simulink model "ARAI_Academy"  (R2020a)
settings: Solver=FixedStepDiscrete  StartTime=0.0  StopTime=10.0  FixedStep=0.02  RelTol=1e-3
InitFcn:
  | mbd_s32k_consistency_checks(bdroot(gcs));
undefined symbols (not defined in the file): Cells_in_Series, LQFP, Temp_in_Series, ts
libraries: hdlsllib x280, mbd_s32k1xx_ec_toolbox x39, simulink x3
(part 2 of 3)

== system ARAI_Academy/Subsystem16/Subsystem12 ==
  In1 : Inport
  Data Type Conversion : DataTypeConversion  OutDataTypeStr=int16
  Demux : Demux  Outputs=8
  Mux : Mux  Inputs=8
  Subsystem : Subsystem
  Subsystem1 : Subsystem
  Subsystem2 : Subsystem
  Subsystem3 : Subsystem
  Subsystem4 : Subsystem
  Subsystem5 : Subsystem
  Subsystem7 : Subsystem
  Subsystem8 : Subsystem
  MO_CT_FLT : Outport
  wires:
  In1/1 -> Data Type Conversion/1
  Demux/1 -> Subsystem/1(u)
  Demux/2 -> Subsystem1/1(u)
  Demux/3 -> Subsystem2/1(u)
  Demux/4 -> Subsystem3/1(u)
  Demux/5 -> Subsystem4/1(u)
  Demux/6 -> Subsystem5/1(u)
  Demux/7 -> Subsystem7/1(u)
  Demux/8 -> Subsystem8/1(u)
  Subsystem/1(Out1) -> Mux/1
  Subsystem1/1(Out1) -> Mux/2
  Subsystem2/1(Out1) -> Mux/3
  Subsystem3/1(Out1) -> Mux/4
  Subsystem4/1(Out1) -> Mux/5
  Subsystem5/1(Out1) -> Mux/6
  Subsystem7/1(Out1) -> Mux/7
  Subsystem8/1(Out1) -> Mux/8
  Mux/1 -> MO_CT_FLT/1
  Data Type Conversion/1 -> Demux/1

== system ARAI_Academy/Subsystem17/Subsystem1 ==
  In1 : Inport
  Bit Slice : hdlsllib/Logic and Bit Operations/Bit Slice  lidx=15  ridx=8
      settings: SourceProductBaseCode=SL
  Bit Slice1 : hdlsllib/Logic and Bit Operations/Bit Slice  lidx=7  ridx=0
      settings: SourceProductBaseCode=SL
  Data Type Conversion : DataTypeConversion  OutDataTypeStr=uint16
  Mux : Mux  Inputs=2
  MO_MaxCellV : Outport
  wires:
  Data Type Conversion/1 -> Bit Slice/1, Bit Slice1/1
  Bit Slice/1 -> Mux/1
  Bit Slice1/1 -> Mux/2
  Mux/1 -> MO_MaxCellV/1  "MaxCellV"
  In1/1 -> Data Type Conversion/1

== system ARAI_Academy/Subsystem17/Subsystem9 ==
  HI_ICT_Raw : Inport
  Bit Slice : hdlsllib/Logic and Bit Operations/Bit Slice  lidx=15  ridx=8
      settings: SourceProductBaseCode=SL
  Bit Slice1 : hdlsllib/Logic and Bit Operations/Bit Slice  lidx=7  ridx=0
      settings: SourceProductBaseCode=SL
  Mux : Mux  Inputs=2
  MO_ICT : Outport
  wires:
  Mux/1 -> MO_ICT/1
  Bit Slice1/1 -> Mux/2
  HI_ICT_Raw/1 -> Bit Slice/1, Bit Slice1/1
  Bit Slice/1 -> Mux/1

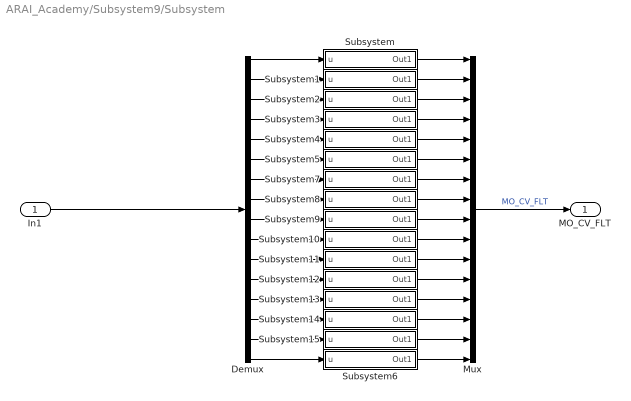
== system ARAI_Academy/Subsystem9/Subsystem ==
  In1 : Inport
  Demux : Demux  Outputs=16
  Mux : Mux  Inputs=16
  Subsystem : Subsystem
  Subsystem1 : Subsystem
  Subsystem10 : Subsystem
  Subsystem11 : Subsystem
  Subsystem12 : Subsystem
  Subsystem13 : Subsystem
  Subsystem14 : Subsystem
  Subsystem15 : Subsystem
  Subsystem2 : Subsystem
  Subsystem3 : Subsystem
  Subsystem4 : Subsystem
  Subsystem5 : Subsystem
  Subsystem6 : Subsystem
  Subsystem7 : Subsystem
  Subsystem8 : Subsystem
  Subsystem9 : Subsystem
  MO_CV_FLT : Outport
  wires:
  In1/1 -> Demux/1
  Demux/1 -> Subsystem/1(u)
  Demux/16 -> Subsystem6/1(u)
  Demux/2 -> Subsystem1/1(u)
  Demux/3 -> Subsystem2/1(u)
  Demux/4 -> Subsystem3/1(u)
  Demux/5 -> Subsystem4/1(u)
  Demux/6 -> Subsystem5/1(u)
  Demux/7 -> Subsystem7/1(u)
  Demux/8 -> Subsystem8/1(u)
  Demux/9 -> Subsystem9/1(u)
  Demux/10 -> Subsystem10/1(u)
  Demux/11 -> Subsystem11/1(u)
  Demux/12 -> Subsystem12/1(u)
  Demux/13 -> Subsystem13/1(u)
  Demux/14 -> Subsystem14/1(u)
  Demux/15 -> Subsystem15/1(u)
  Subsystem/1(Out1) -> Mux/1
  Subsystem1/1(Out1) -> Mux/2
  Subsystem2/1(Out1) -> Mux/3
  Subsystem3/1(Out1) -> Mux/4
  Subsystem4/1(Out1) -> Mux/5
  Subsystem5/1(Out1) -> Mux/6
  Subsystem7/1(Out1) -> Mux/7
  Subsystem8/1(Out1) -> Mux/8
  Subsystem9/1(Out1) -> Mux/9
  Subsystem10/1(Out1) -> Mux/10
  Subsystem11/1(Out1) -> Mux/11
  Subsystem12/1(Out1) -> Mux/12
  Subsystem13/1(Out1) -> Mux/13
  Subsystem14/1(Out1) -> Mux/14
  Subsystem15/1(Out1) -> Mux/15
  Subsystem6/1(Out1) -> Mux/16
  Mux/1 -> MO_CV_FLT/1  "MO_CV_FLT"

== system ARAI_Academy/TNS/ADC ==
  ADC_01 : Subsystem
  ADC_02 : Subsystem

== system ARAI_Academy/TNS/CAN ==
  CAN_01 : Subsystem

== system ARAI_Academy/TNS/I2C ==
  RTC/EEPROM : Subsystem

== system ARAI_Academy/TNS/System Outputs ==

== system ARAI_Academy/AFE_IN_SYS/If Action Subsystem/Subsystem ==
  Constant10 : Constant  Value=8  OutDataTypeStr=uint16  SampleTime=-1
  Constant11 : Constant  Value=32  OutDataTypeStr=uint32  SampleTime=-1
  Constant3 : Constant  Value=0x14  OutDataTypeStr=uint8  SampleTime=-1
  Constant8 : Constant  Value=true  OutDataTypeStr=Inherit: Inherit via back propagation  SampleTime=-1
  LPI2C_Master_Multi_Transfer : mbd_s32k1xx_ec_toolbox/Communication Blocks/I2C Blocks/LPI2C_Master_Multi_Transfer  instance=0  xfermode=Blocking  Timeout=3  delay_between_transfers=0  is10bit=off
  Out1 : Outport  PortDimensions=32
  wires:
  Constant10/1 -> LPI2C_Master_Multi_Transfer/3
  Constant3/1 -> LPI2C_Master_Multi_Transfer/1
  Constant8/1 -> LPI2C_Master_Multi_Transfer/2
  Constant11/1 -> LPI2C_Master_Multi_Transfer/4
  LPI2C_Master_Multi_Transfer/1 -> Out1/1

== system ARAI_Academy/AFE_IN_SYS/If Action Subsystem1/Subsystem ==
  Constant12 : Constant  Value=0x6A  OutDataTypeStr=uint8
  Constant13 : Constant  Value=true  OutDataTypeStr=Inherit: Inherit via back propagation
  Constant14 : Constant  Value=8  OutDataTypeStr=uint16
  Constant18 : Constant  Value=18  OutDataTypeStr=uint32
  LPI2C_Master_Multi_Transfer1 : mbd_s32k1xx_ec_toolbox/Communication Blocks/I2C Blocks/LPI2C_Master_Multi_Transfer  instance=0  xfermode=Blocking  Timeout=3  delay_between_transfers=0  is10bit=off
  Out1 : Outport  OutDataTypeStr=uint8  PortDimensions=18
  wires:
  Constant13/1 -> LPI2C_Master_Multi_Transfer1/2
  Constant18/1 -> LPI2C_Master_Multi_Transfer1/4
  LPI2C_Master_Multi_Transfer1/1 -> Out1/1
  Constant14/1 -> LPI2C_Master_Multi_Transfer1/3
  Constant12/1 -> LPI2C_Master_Multi_Transfer1/1

== system ARAI_Academy/AFE_IN_SYS/Subsystem1/Subsystem ==
  In1 : Inport  PortDimensions=2
  Bit Concat : hdlsllib/Logic and Bit Operations/Bit Concat  numInputs=2
  Demux : Demux  Outputs=2
  y : Outport
  wires:
  Demux/2 -> Bit Concat/2
  Demux/1 -> Bit Concat/1
  Bit Concat/1 -> y/1
  In1/1 -> Demux/1

== system ARAI_Academy/AFE_IN_SYS/Subsystem2/Subsystem ==
  In1 : Inport  PortDimensions=2
  Bit Concat : hdlsllib/Logic and Bit Operations/Bit Concat  numInputs=2
  Demux : Demux  Outputs=2
  y : Outport
  wires:
  Demux/2 -> Bit Concat/1
  Demux/1 -> Bit Concat/2
  Bit Concat/1 -> y/1
  In1/1 -> Demux/1

== system ARAI_Academy/AFE_IN_SYS/Subsystem3/Subsystem ==
  In1 : Inport  PortDimensions=2
  Bit Concat : hdlsllib/Logic and Bit Operations/Bit Concat  numInputs=2
  Demux : Demux  Outputs=2
  y : Outport
  wires:
  Demux/2 -> Bit Concat/1
  Demux/1 -> Bit Concat/2
  Bit Concat/1 -> y/1
  In1/1 -> Demux/1

== system ARAI_Academy/Subsystem10/Subsystem/Subsystem ==
  u : Inport
  Bit Slice : hdlsllib/Logic and Bit Operations/Bit Slice  lidx=15  ridx=8
      settings: SourceProductBaseCode=SL
  Bit Slice1 : hdlsllib/Logic and Bit Operations/Bit Slice  lidx=7  ridx=0
      settings: SourceProductBaseCode=SL
  Mux : Mux  Inputs=2
  Out1 : Outport
  wires:
  Bit Slice/1 -> Mux/1
  u/1 -> Bit Slice/1, Bit Slice1/1
  Bit Slice1/1 -> Mux/2
  Mux/1 -> Out1/1

== system ARAI_Academy/Subsystem10/Subsystem/Subsystem1 ==
  u : Inport
  Bit Slice : hdlsllib/Logic and Bit Operations/Bit Slice  lidx=15  ridx=8
      settings: SourceProductBaseCode=SL
  Bit Slice1 : hdlsllib/Logic and Bit Operations/Bit Slice  lidx=7  ridx=0
      settings: SourceProductBaseCode=SL
  Mux : Mux  Inputs=2
  Out1 : Outport
  wires:
  Bit Slice/1 -> Mux/1
  u/1 -> Bit Slice/1, Bit Slice1/1
  Bit Slice1/1 -> Mux/2
  Mux/1 -> Out1/1

== system ARAI_Academy/Subsystem10/Subsystem/Subsystem10 ==
  u : Inport
  Bit Slice : hdlsllib/Logic and Bit Operations/Bit Slice  lidx=15  ridx=8
      settings: SourceProductBaseCode=SL
  Bit Slice1 : hdlsllib/Logic and Bit Operations/Bit Slice  lidx=7  ridx=0
      settings: SourceProductBaseCode=SL
  Mux : Mux  Inputs=2
  Out1 : Outport
  wires:
  Bit Slice/1 -> Mux/1
  u/1 -> Bit Slice/1, Bit Slice1/1
  Bit Slice1/1 -> Mux/2
  Mux/1 -> Out1/1

== system ARAI_Academy/Subsystem10/Subsystem/Subsystem11 ==
  u : Inport
  Bit Slice : hdlsllib/Logic and Bit Operations/Bit Slice  lidx=15  ridx=8
      settings: SourceProductBaseCode=SL
  Bit Slice1 : hdlsllib/Logic and Bit Operations/Bit Slice  lidx=7  ridx=0
      settings: SourceProductBaseCode=SL
  Mux : Mux  Inputs=2
  Out1 : Outport
  wires:
  Mux/1 -> Out1/1
  Bit Slice1/1 -> Mux/2
  u/1 -> Bit Slice1/1, Bit Slice/1
  Bit Slice/1 -> Mux/1

== system ARAI_Academy/Subsystem10/Subsystem/Subsystem12 ==
  u : Inport
  Bit Slice : hdlsllib/Logic and Bit Operations/Bit Slice  lidx=15  ridx=8
      settings: SourceProductBaseCode=SL
  Bit Slice1 : hdlsllib/Logic and Bit Operations/Bit Slice  lidx=7  ridx=0
      settings: SourceProductBaseCode=SL
  Mux : Mux  Inputs=2
  Out1 : Outport
  wires:
  Bit Slice/1 -> Mux/1
  u/1 -> Bit Slice/1, Bit Slice1/1
  Bit Slice1/1 -> Mux/2
  Mux/1 -> Out1/1

== system ARAI_Academy/Subsystem10/Subsystem/Subsystem13 ==
  u : Inport
  Bit Slice : hdlsllib/Logic and Bit Operations/Bit Slice  lidx=15  ridx=8
      settings: SourceProductBaseCode=SL
  Bit Slice1 : hdlsllib/Logic and Bit Operations/Bit Slice  lidx=7  ridx=0
      settings: SourceProductBaseCode=SL
  Mux : Mux  Inputs=2
  Out1 : Outport
  wires:
  Mux/1 -> Out1/1
  Bit Slice1/1 -> Mux/2
  u/1 -> Bit Slice1/1, Bit Slice/1
  Bit Slice/1 -> Mux/1

== system ARAI_Academy/Subsystem10/Subsystem/Subsystem14 ==
  u : Inport
  Bit Slice : hdlsllib/Logic and Bit Operations/Bit Slice  lidx=15  ridx=8
      settings: SourceProductBaseCode=SL
  Bit Slice1 : hdlsllib/Logic and Bit Operations/Bit Slice  lidx=7  ridx=0
      settings: SourceProductBaseCode=SL
  Mux : Mux  Inputs=2
  Out1 : Outport
  wires:
  Bit Slice/1 -> Mux/1
  u/1 -> Bit Slice/1, Bit Slice1/1
  Bit Slice1/1 -> Mux/2
  Mux/1 -> Out1/1

== system ARAI_Academy/Subsystem10/Subsystem/Subsystem15 ==
  u : Inport
  Bit Slice : hdlsllib/Logic and Bit Operations/Bit Slice  lidx=15  ridx=8
      settings: SourceProductBaseCode=SL
  Bit Slice1 : hdlsllib/Logic and Bit Operations/Bit Slice  lidx=7  ridx=0
      settings: SourceProductBaseCode=SL
  Mux : Mux  Inputs=2
  Out1 : Outport
  wires:
  Mux/1 -> Out1/1
  Bit Slice1/1 -> Mux/2
  u/1 -> Bit Slice1/1, Bit Slice/1
  Bit Slice/1 -> Mux/1

== system ARAI_Academy/Subsystem10/Subsystem/Subsystem2 ==
  u : Inport
  Bit Slice : hdlsllib/Logic and Bit Operations/Bit Slice  lidx=15  ridx=8
      settings: SourceProductBaseCode=SL
  Bit Slice1 : hdlsllib/Logic and Bit Operations/Bit Slice  lidx=7  ridx=0
      settings: SourceProductBaseCode=SL
  Mux : Mux  Inputs=2
  Out1 : Outport
  wires:
  Bit Slice/1 -> Mux/1
  u/1 -> Bit Slice/1, Bit Slice1/1
  Bit Slice1/1 -> Mux/2
  Mux/1 -> Out1/1

== system ARAI_Academy/Subsystem10/Subsystem/Subsystem3 ==
  u : Inport
  Bit Slice : hdlsllib/Logic and Bit Operations/Bit Slice  lidx=15  ridx=8
      settings: SourceProductBaseCode=SL
  Bit Slice1 : hdlsllib/Logic and Bit Operations/Bit Slice  lidx=7  ridx=0
      settings: SourceProductBaseCode=SL
  Mux : Mux  Inputs=2
  Out1 : Outport
  wires:
  Bit Slice/1 -> Mux/1
  u/1 -> Bit Slice/1, Bit Slice1/1
  Bit Slice1/1 -> Mux/2
  Mux/1 -> Out1/1

== system ARAI_Academy/Subsystem10/Subsystem/Subsystem4 ==
  u : Inport
  Bit Slice : hdlsllib/Logic and Bit Operations/Bit Slice  lidx=15  ridx=8
      settings: SourceProductBaseCode=SL
  Bit Slice1 : hdlsllib/Logic and Bit Operations/Bit Slice  lidx=7  ridx=0
      settings: SourceProductBaseCode=SL
  Mux : Mux  Inputs=2
  Out1 : Outport
  wires:
  Bit Slice/1 -> Mux/1
  u/1 -> Bit Slice/1, Bit Slice1/1
  Bit Slice1/1 -> Mux/2
  Mux/1 -> Out1/1

== system ARAI_Academy/Subsystem10/Subsystem/Subsystem5 ==
  u : Inport
  Bit Slice : hdlsllib/Logic and Bit Operations/Bit Slice  lidx=15  ridx=8
      settings: SourceProductBaseCode=SL
  Bit Slice1 : hdlsllib/Logic and Bit Operations/Bit Slice  lidx=7  ridx=0
      settings: SourceProductBaseCode=SL
  Mux : Mux  Inputs=2
  Out1 : Outport
  wires:
  Bit Slice/1 -> Mux/1
  u/1 -> Bit Slice/1, Bit Slice1/1
  Bit Slice1/1 -> Mux/2
  Mux/1 -> Out1/1

== system ARAI_Academy/Subsystem10/Subsystem/Subsystem6 ==
  u : Inport
  Bit Slice : hdlsllib/Logic and Bit Operations/Bit Slice  lidx=15  ridx=8
      settings: SourceProductBaseCode=SL
  Bit Slice1 : hdlsllib/Logic and Bit Operations/Bit Slice  lidx=7  ridx=0
      settings: SourceProductBaseCode=SL
  Mux : Mux  Inputs=2
  Out1 : Outport
  wires:
  Bit Slice/1 -> Mux/1
  u/1 -> Bit Slice/1, Bit Slice1/1
  Bit Slice1/1 -> Mux/2
  Mux/1 -> Out1/1

== system ARAI_Academy/Subsystem10/Subsystem/Subsystem7 ==
  u : Inport
  Bit Slice : hdlsllib/Logic and Bit Operations/Bit Slice  lidx=15  ridx=8
      settings: SourceProductBaseCode=SL
  Bit Slice1 : hdlsllib/Logic and Bit Operations/Bit Slice  lidx=7  ridx=0
      settings: SourceProductBaseCode=SL
  Mux : Mux  Inputs=2
  Out1 : Outport
  wires:
  Mux/1 -> Out1/1
  Bit Slice1/1 -> Mux/2
  u/1 -> Bit Slice1/1, Bit Slice/1
  Bit Slice/1 -> Mux/1

== system ARAI_Academy/Subsystem10/Subsystem/Subsystem8 ==
  u : Inport
  Bit Slice : hdlsllib/Logic and Bit Operations/Bit Slice  lidx=15  ridx=8
      settings: SourceProductBaseCode=SL
  Bit Slice1 : hdlsllib/Logic and Bit Operations/Bit Slice  lidx=7  ridx=0
      settings: SourceProductBaseCode=SL
  Mux : Mux  Inputs=2
  Out1 : Outport
  wires:
  Bit Slice/1 -> Mux/1
  u/1 -> Bit Slice/1, Bit Slice1/1
  Bit Slice1/1 -> Mux/2
  Mux/1 -> Out1/1

== system ARAI_Academy/Subsystem10/Subsystem/Subsystem9 ==
  u : Inport
  Bit Slice : hdlsllib/Logic and Bit Operations/Bit Slice  lidx=15  ridx=8
      settings: SourceProductBaseCode=SL
  Bit Slice1 : hdlsllib/Logic and Bit Operations/Bit Slice  lidx=7  ridx=0
      settings: SourceProductBaseCode=SL
  Mux : Mux  Inputs=2
  Out1 : Outport
  wires:
  Mux/1 -> Out1/1
  Bit Slice1/1 -> Mux/2
  u/1 -> Bit Slice1/1, Bit Slice/1
  Bit Slice/1 -> Mux/1

== system ARAI_Academy/Subsystem11/Subsystem/Subsystem ==
  u : Inport
  Bit Slice : hdlsllib/Logic and Bit Operations/Bit Slice  lidx=15  ridx=8
      settings: SourceProductBaseCode=SL
  Bit Slice1 : hdlsllib/Logic and Bit Operations/Bit Slice  lidx=7  ridx=0
      settings: SourceProductBaseCode=SL
  Mux : Mux  Inputs=2
  Out1 : Outport
  wires:
  Bit Slice/1 -> Mux/1
  u/1 -> Bit Slice/1, Bit Slice1/1
  Bit Slice1/1 -> Mux/2
  Mux/1 -> Out1/1

== system ARAI_Academy/Subsystem11/Subsystem/Subsystem1 ==
  u : Inport
  Bit Slice : hdlsllib/Logic and Bit Operations/Bit Slice  lidx=15  ridx=8
      settings: SourceProductBaseCode=SL
  Bit Slice1 : hdlsllib/Logic and Bit Operations/Bit Slice  lidx=7  ridx=0
      settings: SourceProductBaseCode=SL
  Mux : Mux  Inputs=2
  Out1 : Outport
  wires:
  Bit Slice/1 -> Mux/1
  u/1 -> Bit Slice/1, Bit Slice1/1
  Bit Slice1/1 -> Mux/2
  Mux/1 -> Out1/1

== system ARAI_Academy/Subsystem11/Subsystem/Subsystem10 ==
  u : Inport
  Bit Slice : hdlsllib/Logic and Bit Operations/Bit Slice  lidx=15  ridx=8
      settings: SourceProductBaseCode=SL
  Bit Slice1 : hdlsllib/Logic and Bit Operations/Bit Slice  lidx=7  ridx=0
      settings: SourceProductBaseCode=SL
  Mux : Mux  Inputs=2
  Out1 : Outport
  wires:
  Bit Slice/1 -> Mux/1
  u/1 -> Bit Slice/1, Bit Slice1/1
  Bit Slice1/1 -> Mux/2
  Mux/1 -> Out1/1

== system ARAI_Academy/Subsystem11/Subsystem/Subsystem11 ==
  u : Inport
  Bit Slice : hdlsllib/Logic and Bit Operations/Bit Slice  lidx=15  ridx=8
      settings: SourceProductBaseCode=SL
  Bit Slice1 : hdlsllib/Logic and Bit Operations/Bit Slice  lidx=7  ridx=0
      settings: SourceProductBaseCode=SL
  Mux : Mux  Inputs=2
  Out1 : Outport
  wires:
  Mux/1 -> Out1/1
  Bit Slice1/1 -> Mux/2
  u/1 -> Bit Slice1/1, Bit Slice/1
  Bit Slice/1 -> Mux/1

== system ARAI_Academy/Subsystem11/Subsystem/Subsystem12 ==
  u : Inport
  Bit Slice : hdlsllib/Logic and Bit Operations/Bit Slice  lidx=15  ridx=8
      settings: SourceProductBaseCode=SL
  Bit Slice1 : hdlsllib/Logic and Bit Operations/Bit Slice  lidx=7  ridx=0
      settings: SourceProductBaseCode=SL
  Mux : Mux  Inputs=2
  Out1 : Outport
  wires:
  Bit Slice/1 -> Mux/1
  u/1 -> Bit Slice/1, Bit Slice1/1
  Bit Slice1/1 -> Mux/2
  Mux/1 -> Out1/1

== system ARAI_Academy/Subsystem11/Subsystem/Subsystem13 ==
  u : Inport
  Bit Slice : hdlsllib/Logic and Bit Operations/Bit Slice  lidx=15  ridx=8
      settings: SourceProductBaseCode=SL
  Bit Slice1 : hdlsllib/Logic and Bit Operations/Bit Slice  lidx=7  ridx=0
      settings: SourceProductBaseCode=SL
  Mux : Mux  Inputs=2
  Out1 : Outport
  wires:
  Mux/1 -> Out1/1
  Bit Slice1/1 -> Mux/2
  u/1 -> Bit Slice1/1, Bit Slice/1
  Bit Slice/1 -> Mux/1

== system ARAI_Academy/Subsystem11/Subsystem/Subsystem14 ==
  u : Inport
  Bit Slice : hdlsllib/Logic and Bit Operations/Bit Slice  lidx=15  ridx=8
      settings: SourceProductBaseCode=SL
  Bit Slice1 : hdlsllib/Logic and Bit Operations/Bit Slice  lidx=7  ridx=0
      settings: SourceProductBaseCode=SL
  Mux : Mux  Inputs=2
  Out1 : Outport
  wires:
  Bit Slice/1 -> Mux/1
  u/1 -> Bit Slice/1, Bit Slice1/1
  Bit Slice1/1 -> Mux/2
  Mux/1 -> Out1/1

== system ARAI_Academy/Subsystem11/Subsystem/Subsystem15 ==
  u : Inport
  Bit Slice : hdlsllib/Logic and Bit Operations/Bit Slice  lidx=15  ridx=8
      settings: SourceProductBaseCode=SL
  Bit Slice1 : hdlsllib/Logic and Bit Operations/Bit Slice  lidx=7  ridx=0
      settings: SourceProductBaseCode=SL
  Mux : Mux  Inputs=2
  Out1 : Outport
  wires:
  Mux/1 -> Out1/1
  Bit Slice1/1 -> Mux/2
  u/1 -> Bit Slice1/1, Bit Slice/1
  Bit Slice/1 -> Mux/1

== system ARAI_Academy/Subsystem11/Subsystem/Subsystem2 ==
  u : Inport
  Bit Slice : hdlsllib/Logic and Bit Operations/Bit Slice  lidx=15  ridx=8
      settings: SourceProductBaseCode=SL
  Bit Slice1 : hdlsllib/Logic and Bit Operations/Bit Slice  lidx=7  ridx=0
      settings: SourceProductBaseCode=SL
  Mux : Mux  Inputs=2
  Out1 : Outport
  wires:
  Bit Slice/1 -> Mux/1
  u/1 -> Bit Slice/1, Bit Slice1/1
  Bit Slice1/1 -> Mux/2
  Mux/1 -> Out1/1

== system ARAI_Academy/Subsystem11/Subsystem/Subsystem3 ==
  u : Inport
  Bit Slice : hdlsllib/Logic and Bit Operations/Bit Slice  lidx=15  ridx=8
      settings: SourceProductBaseCode=SL
  Bit Slice1 : hdlsllib/Logic and Bit Operations/Bit Slice  lidx=7  ridx=0
      settings: SourceProductBaseCode=SL
  Mux : Mux  Inputs=2
  Out1 : Outport
  wires:
  Bit Slice/1 -> Mux/1
  u/1 -> Bit Slice/1, Bit Slice1/1
  Bit Slice1/1 -> Mux/2
  Mux/1 -> Out1/1

== system ARAI_Academy/Subsystem11/Subsystem/Subsystem4 ==
  u : Inport
  Bit Slice : hdlsllib/Logic and Bit Operations/Bit Slice  lidx=15  ridx=8
      settings: SourceProductBaseCode=SL
  Bit Slice1 : hdlsllib/Logic and Bit Operations/Bit Slice  lidx=7  ridx=0
      settings: SourceProductBaseCode=SL
  Mux : Mux  Inputs=2
  Out1 : Outport
  wires:
  Bit Slice/1 -> Mux/1
  u/1 -> Bit Slice/1, Bit Slice1/1
  Bit Slice1/1 -> Mux/2
  Mux/1 -> Out1/1

== system ARAI_Academy/Subsystem11/Subsystem/Subsystem5 ==
  u : Inport
  Bit Slice : hdlsllib/Logic and Bit Operations/Bit Slice  lidx=15  ridx=8
      settings: SourceProductBaseCode=SL
  Bit Slice1 : hdlsllib/Logic and Bit Operations/Bit Slice  lidx=7  ridx=0
      settings: SourceProductBaseCode=SL
  Mux : Mux  Inputs=2
  Out1 : Outport
  wires:
  Bit Slice/1 -> Mux/1
  u/1 -> Bit Slice/1, Bit Slice1/1
  Bit Slice1/1 -> Mux/2
  Mux/1 -> Out1/1

== system ARAI_Academy/Subsystem11/Subsystem/Subsystem6 ==
  u : Inport
  Bit Slice : hdlsllib/Logic and Bit Operations/Bit Slice  lidx=15  ridx=8
      settings: SourceProductBaseCode=SL
  Bit Slice1 : hdlsllib/Logic and Bit Operations/Bit Slice  lidx=7  ridx=0
      settings: SourceProductBaseCode=SL
  Mux : Mux  Inputs=2
  Out1 : Outport
  wires:
  Bit Slice/1 -> Mux/1
  u/1 -> Bit Slice/1, Bit Slice1/1
  Bit Slice1/1 -> Mux/2
  Mux/1 -> Out1/1

== system ARAI_Academy/Subsystem11/Subsystem/Subsystem7 ==
  u : Inport
  Bit Slice : hdlsllib/Logic and Bit Operations/Bit Slice  lidx=15  ridx=8
      settings: SourceProductBaseCode=SL
  Bit Slice1 : hdlsllib/Logic and Bit Operations/Bit Slice  lidx=7  ridx=0
      settings: SourceProductBaseCode=SL
  Mux : Mux  Inputs=2
  Out1 : Outport
  wires:
  Mux/1 -> Out1/1
  Bit Slice1/1 -> Mux/2
  u/1 -> Bit Slice1/1, Bit Slice/1
  Bit Slice/1 -> Mux/1

== system ARAI_Academy/Subsystem11/Subsystem/Subsystem8 ==
  u : Inport
  Bit Slice : hdlsllib/Logic and Bit Operations/Bit Slice  lidx=15  ridx=8
      settings: SourceProductBaseCode=SL
  Bit Slice1 : hdlsllib/Logic and Bit Operations/Bit Slice  lidx=7  ridx=0
      settings: SourceProductBaseCode=SL
  Mux : Mux  Inputs=2
  Out1 : Outport
  wires:
  Bit Slice/1 -> Mux/1
  u/1 -> Bit Slice/1, Bit Slice1/1
  Bit Slice1/1 -> Mux/2
  Mux/1 -> Out1/1

== system ARAI_Academy/Subsystem11/Subsystem/Subsystem9 ==
  u : Inport
  Bit Slice : hdlsllib/Logic and Bit Operations/Bit Slice  lidx=15  ridx=8
      settings: SourceProductBaseCode=SL
  Bit Slice1 : hdlsllib/Logic and Bit Operations/Bit Slice  lidx=7  ridx=0
      settings: SourceProductBaseCode=SL
  Mux : Mux  Inputs=2
  Out1 : Outport
  wires:
  Mux/1 -> Out1/1
  Bit Slice1/1 -> Mux/2
  u/1 -> Bit Slice1/1, Bit Slice/1
  Bit Slice/1 -> Mux/1

== system ARAI_Academy/Subsystem12/Subsystem/Subsystem ==
  u : Inport
  Bit Slice : hdlsllib/Logic and Bit Operations/Bit Slice  lidx=15  ridx=8
      settings: SourceProductBaseCode=SL
  Bit Slice1 : hdlsllib/Logic and Bit Operations/Bit Slice  lidx=7  ridx=0
      settings: SourceProductBaseCode=SL
  Mux : Mux  Inputs=2
  Out1 : Outport
  wires:
  Bit Slice/1 -> Mux/1
  u/1 -> Bit Slice/1, Bit Slice1/1
  Bit Slice1/1 -> Mux/2
  Mux/1 -> Out1/1

== system ARAI_Academy/Subsystem12/Subsystem/Subsystem1 ==
  u : Inport
  Bit Slice : hdlsllib/Logic and Bit Operations/Bit Slice  lidx=15  ridx=8
      settings: SourceProductBaseCode=SL
  Bit Slice1 : hdlsllib/Logic and Bit Operations/Bit Slice  lidx=7  ridx=0
      settings: SourceProductBaseCode=SL
  Mux : Mux  Inputs=2
  Out1 : Outport
  wires:
  Bit Slice/1 -> Mux/1
  u/1 -> Bit Slice/1, Bit Slice1/1
  Bit Slice1/1 -> Mux/2
  Mux/1 -> Out1/1

== system ARAI_Academy/Subsystem12/Subsystem/Subsystem10 ==
  u : Inport
  Bit Slice : hdlsllib/Logic and Bit Operations/Bit Slice  lidx=15  ridx=8
      settings: SourceProductBaseCode=SL
  Bit Slice1 : hdlsllib/Logic and Bit Operations/Bit Slice  lidx=7  ridx=0
      settings: SourceProductBaseCode=SL
  Mux : Mux  Inputs=2
  Out1 : Outport
  wires:
  Bit Slice/1 -> Mux/1
  u/1 -> Bit Slice/1, Bit Slice1/1
  Bit Slice1/1 -> Mux/2
  Mux/1 -> Out1/1

== system ARAI_Academy/Subsystem12/Subsystem/Subsystem11 ==
  u : Inport
  Bit Slice : hdlsllib/Logic and Bit Operations/Bit Slice  lidx=15  ridx=8
      settings: SourceProductBaseCode=SL
  Bit Slice1 : hdlsllib/Logic and Bit Operations/Bit Slice  lidx=7  ridx=0
      settings: SourceProductBaseCode=SL
  Mux : Mux  Inputs=2
  Out1 : Outport
  wires:
  Mux/1 -> Out1/1
  Bit Slice1/1 -> Mux/2
  u/1 -> Bit Slice1/1, Bit Slice/1
  Bit Slice/1 -> Mux/1

== system ARAI_Academy/Subsystem12/Subsystem/Subsystem12 ==
  u : Inport
  Bit Slice : hdlsllib/Logic and Bit Operations/Bit Slice  lidx=15  ridx=8
      settings: SourceProductBaseCode=SL
  Bit Slice1 : hdlsllib/Logic and Bit Operations/Bit Slice  lidx=7  ridx=0
      settings: SourceProductBaseCode=SL
  Mux : Mux  Inputs=2
  Out1 : Outport
  wires:
  Bit Slice/1 -> Mux/1
  u/1 -> Bit Slice/1, Bit Slice1/1
  Bit Slice1/1 -> Mux/2
  Mux/1 -> Out1/1

== system ARAI_Academy/Subsystem12/Subsystem/Subsystem13 ==
  u : Inport
  Bit Slice : hdlsllib/Logic and Bit Operations/Bit Slice  lidx=15  ridx=8
      settings: SourceProductBaseCode=SL
  Bit Slice1 : hdlsllib/Logic and Bit Operations/Bit Slice  lidx=7  ridx=0
      settings: SourceProductBaseCode=SL
  Mux : Mux  Inputs=2
  Out1 : Outport
  wires:
  Mux/1 -> Out1/1
  Bit Slice1/1 -> Mux/2
  u/1 -> Bit Slice1/1, Bit Slice/1
  Bit Slice/1 -> Mux/1

== system ARAI_Academy/Subsystem12/Subsystem/Subsystem14 ==
  u : Inport
  Bit Slice : hdlsllib/Logic and Bit Operations/Bit Slice  lidx=15  ridx=8
      settings: SourceProductBaseCode=SL
  Bit Slice1 : hdlsllib/Logic and Bit Operations/Bit Slice  lidx=7  ridx=0
      settings: SourceProductBaseCode=SL
  Mux : Mux  Inputs=2
  Out1 : Outport
  wires:
  Bit Slice/1 -> Mux/1
  u/1 -> Bit Slice/1, Bit Slice1/1
  Bit Slice1/1 -> Mux/2
  Mux/1 -> Out1/1

== system ARAI_Academy/Subsystem12/Subsystem/Subsystem15 ==
  u : Inport
  Bit Slice : hdlsllib/Logic and Bit Operations/Bit Slice  lidx=15  ridx=8
      settings: SourceProductBaseCode=SL
  Bit Slice1 : hdlsllib/Logic and Bit Operations/Bit Slice  lidx=7  ridx=0
      settings: SourceProductBaseCode=SL
  Mux : Mux  Inputs=2
  Out1 : Outport
  wires:
  Mux/1 -> Out1/1
  Bit Slice1/1 -> Mux/2
  u/1 -> Bit Slice1/1, Bit Slice/1
  Bit Slice/1 -> Mux/1

== system ARAI_Academy/Subsystem12/Subsystem/Subsystem2 ==
  u : Inport
  Bit Slice : hdlsllib/Logic and Bit Operations/Bit Slice  lidx=15  ridx=8
      settings: SourceProductBaseCode=SL
  Bit Slice1 : hdlsllib/Logic and Bit Operations/Bit Slice  lidx=7  ridx=0
      settings: SourceProductBaseCode=SL
  Mux : Mux  Inputs=2
  Out1 : Outport
  wires:
  Bit Slice/1 -> Mux/1
  u/1 -> Bit Slice/1, Bit Slice1/1
  Bit Slice1/1 -> Mux/2
  Mux/1 -> Out1/1

== system ARAI_Academy/Subsystem12/Subsystem/Subsystem3 ==
  u : Inport
  Bit Slice : hdlsllib/Logic and Bit Operations/Bit Slice  lidx=15  ridx=8
      settings: SourceProductBaseCode=SL
  Bit Slice1 : hdlsllib/Logic and Bit Operations/Bit Slice  lidx=7  ridx=0
      settings: SourceProductBaseCode=SL
  Mux : Mux  Inputs=2
  Out1 : Outport
  wires:
  Bit Slice/1 -> Mux/1
  u/1 -> Bit Slice/1, Bit Slice1/1
  Bit Slice1/1 -> Mux/2
  Mux/1 -> Out1/1

== system ARAI_Academy/Subsystem12/Subsystem/Subsystem4 ==
  u : Inport
  Bit Slice : hdlsllib/Logic and Bit Operations/Bit Slice  lidx=15  ridx=8
      settings: SourceProductBaseCode=SL
  Bit Slice1 : hdlsllib/Logic and Bit Operations/Bit Slice  lidx=7  ridx=0
      settings: SourceProductBaseCode=SL
  Mux : Mux  Inputs=2
  Out1 : Outport
  wires:
  Bit Slice/1 -> Mux/1
  u/1 -> Bit Slice/1, Bit Slice1/1
  Bit Slice1/1 -> Mux/2
  Mux/1 -> Out1/1

== system ARAI_Academy/Subsystem12/Subsystem/Subsystem5 ==
  u : Inport
  Bit Slice : hdlsllib/Logic and Bit Operations/Bit Slice  lidx=15  ridx=8
      settings: SourceProductBaseCode=SL
  Bit Slice1 : hdlsllib/Logic and Bit Operations/Bit Slice  lidx=7  ridx=0
      settings: SourceProductBaseCode=SL
  Mux : Mux  Inputs=2
  Out1 : Outport
  wires:
  Bit Slice/1 -> Mux/1
  u/1 -> Bit Slice/1, Bit Slice1/1
  Bit Slice1/1 -> Mux/2
  Mux/1 -> Out1/1

== system ARAI_Academy/Subsystem12/Subsystem/Subsystem6 ==
  u : Inport
  Bit Slice : hdlsllib/Logic and Bit Operations/Bit Slice  lidx=15  ridx=8
      settings: SourceProductBaseCode=SL
  Bit Slice1 : hdlsllib/Logic and Bit Operations/Bit Slice  lidx=7  ridx=0
      settings: SourceProductBaseCode=SL
  Mux : Mux  Inputs=2
  Out1 : Outport
  wires:
  Bit Slice/1 -> Mux/1
  u/1 -> Bit Slice/1, Bit Slice1/1
  Bit Slice1/1 -> Mux/2
  Mux/1 -> Out1/1

== system ARAI_Academy/Subsystem12/Subsystem/Subsystem7 ==
  u : Inport
  Bit Slice : hdlsllib/Logic and Bit Operations/Bit Slice  lidx=15  ridx=8
      settings: SourceProductBaseCode=SL
  Bit Slice1 : hdlsllib/Logic and Bit Operations/Bit Slice  lidx=7  ridx=0
      settings: SourceProductBaseCode=SL
  Mux : Mux  Inputs=2
  Out1 : Outport
  wires:
  Mux/1 -> Out1/1
  Bit Slice1/1 -> Mux/2
  u/1 -> Bit Slice1/1, Bit Slice/1
  Bit Slice/1 -> Mux/1

== system ARAI_Academy/Subsystem12/Subsystem/Subsystem8 ==
  u : Inport
  Bit Slice : hdlsllib/Logic and Bit Operations/Bit Slice  lidx=15  ridx=8
      settings: SourceProductBaseCode=SL
  Bit Slice1 : hdlsllib/Logic and Bit Operations/Bit Slice  lidx=7  ridx=0
      settings: SourceProductBaseCode=SL
  Mux : Mux  Inputs=2
  Out1 : Outport
  wires:
  Bit Slice/1 -> Mux/1
  u/1 -> Bit Slice/1, Bit Slice1/1
  Bit Slice1/1 -> Mux/2
  Mux/1 -> Out1/1

== system ARAI_Academy/Subsystem12/Subsystem/Subsystem9 ==
  u : Inport
  Bit Slice : hdlsllib/Logic and Bit Operations/Bit Slice  lidx=15  ridx=8
      settings: SourceProductBaseCode=SL
  Bit Slice1 : hdlsllib/Logic and Bit Operations/Bit Slice  lidx=7  ridx=0
      settings: SourceProductBaseCode=SL
  Mux : Mux  Inputs=2
  Out1 : Outport
  wires:
  Mux/1 -> Out1/1
  Bit Slice1/1 -> Mux/2
  u/1 -> Bit Slice1/1, Bit Slice/1
  Bit Slice/1 -> Mux/1

== system ARAI_Academy/Subsystem13/Subsystem/Subsystem ==
  u : Inport
  Bit Slice : hdlsllib/Logic and Bit Operations/Bit Slice  lidx=15  ridx=8
      settings: SourceProductBaseCode=SL
  Bit Slice1 : hdlsllib/Logic and Bit Operations/Bit Slice  lidx=7  ridx=0
      settings: SourceProductBaseCode=SL
  Mux : Mux  Inputs=2
  Out1 : Outport
  wires:
  Bit Slice/1 -> Mux/1
  u/1 -> Bit Slice/1, Bit Slice1/1
  Bit Slice1/1 -> Mux/2
  Mux/1 -> Out1/1

== system ARAI_Academy/Subsystem13/Subsystem/Subsystem1 ==
  u : Inport
  Bit Slice : hdlsllib/Logic and Bit Operations/Bit Slice  lidx=15  ridx=8
      settings: SourceProductBaseCode=SL
  Bit Slice1 : hdlsllib/Logic and Bit Operations/Bit Slice  lidx=7  ridx=0
      settings: SourceProductBaseCode=SL
  Mux : Mux  Inputs=2
  Out1 : Outport
  wires:
  Bit Slice/1 -> Mux/1
  u/1 -> Bit Slice/1, Bit Slice1/1
  Bit Slice1/1 -> Mux/2
  Mux/1 -> Out1/1

== system ARAI_Academy/Subsystem13/Subsystem/Subsystem10 ==
  u : Inport
  Bit Slice : hdlsllib/Logic and Bit Operations/Bit Slice  lidx=15  ridx=8
      settings: SourceProductBaseCode=SL
  Bit Slice1 : hdlsllib/Logic and Bit Operations/Bit Slice  lidx=7  ridx=0
      settings: SourceProductBaseCode=SL
  Mux : Mux  Inputs=2
  Out1 : Outport
  wires:
  Bit Slice/1 -> Mux/1
  u/1 -> Bit Slice/1, Bit Slice1/1
  Bit Slice1/1 -> Mux/2
  Mux/1 -> Out1/1

== system ARAI_Academy/Subsystem13/Subsystem/Subsystem11 ==
  u : Inport
  Bit Slice : hdlsllib/Logic and Bit Operations/Bit Slice  lidx=15  ridx=8
      settings: SourceProductBaseCode=SL
  Bit Slice1 : hdlsllib/Logic and Bit Operations/Bit Slice  lidx=7  ridx=0
      settings: SourceProductBaseCode=SL
  Mux : Mux  Inputs=2
  Out1 : Outport
  wires:
  Mux/1 -> Out1/1
  Bit Slice1/1 -> Mux/2
  u/1 -> Bit Slice1/1, Bit Slice/1
  Bit Slice/1 -> Mux/1

== system ARAI_Academy/Subsystem13/Subsystem/Subsystem12 ==
  u : Inport
  Bit Slice : hdlsllib/Logic and Bit Operations/Bit Slice  lidx=15  ridx=8
      settings: SourceProductBaseCode=SL
  Bit Slice1 : hdlsllib/Logic and Bit Operations/Bit Slice  lidx=7  ridx=0
      settings: SourceProductBaseCode=SL
  Mux : Mux  Inputs=2
  Out1 : Outport
  wires:
  Bit Slice/1 -> Mux/1
  u/1 -> Bit Slice/1, Bit Slice1/1
  Bit Slice1/1 -> Mux/2
  Mux/1 -> Out1/1

== system ARAI_Academy/Subsystem13/Subsystem/Subsystem13 ==
  u : Inport
  Bit Slice : hdlsllib/Logic and Bit Operations/Bit Slice  lidx=15  ridx=8
      settings: SourceProductBaseCode=SL
  Bit Slice1 : hdlsllib/Logic and Bit Operations/Bit Slice  lidx=7  ridx=0
      settings: SourceProductBaseCode=SL
  Mux : Mux  Inputs=2
  Out1 : Outport
  wires:
  Mux/1 -> Out1/1
  Bit Slice1/1 -> Mux/2
  u/1 -> Bit Slice1/1, Bit Slice/1
  Bit Slice/1 -> Mux/1

== system ARAI_Academy/Subsystem13/Subsystem/Subsystem14 ==
  u : Inport
  Bit Slice : hdlsllib/Logic and Bit Operations/Bit Slice  lidx=15  ridx=8
      settings: SourceProductBaseCode=SL
  Bit Slice1 : hdlsllib/Logic and Bit Operations/Bit Slice  lidx=7  ridx=0
      settings: SourceProductBaseCode=SL
  Mux : Mux  Inputs=2
  Out1 : Outport
  wires:
  Bit Slice/1 -> Mux/1
  u/1 -> Bit Slice/1, Bit Slice1/1
  Bit Slice1/1 -> Mux/2
  Mux/1 -> Out1/1

== system ARAI_Academy/Subsystem13/Subsystem/Subsystem15 ==
  u : Inport
  Bit Slice : hdlsllib/Logic and Bit Operations/Bit Slice  lidx=15  ridx=8
      settings: SourceProductBaseCode=SL
  Bit Slice1 : hdlsllib/Logic and Bit Operations/Bit Slice  lidx=7  ridx=0
      settings: SourceProductBaseCode=SL
  Mux : Mux  Inputs=2
  Out1 : Outport
  wires:
  Mux/1 -> Out1/1
  Bit Slice1/1 -> Mux/2
  u/1 -> Bit Slice1/1, Bit Slice/1
  Bit Slice/1 -> Mux/1

== system ARAI_Academy/Subsystem13/Subsystem/Subsystem2 ==
  u : Inport
  Bit Slice : hdlsllib/Logic and Bit Operations/Bit Slice  lidx=15  ridx=8
      settings: SourceProductBaseCode=SL
  Bit Slice1 : hdlsllib/Logic and Bit Operations/Bit Slice  lidx=7  ridx=0
      settings: SourceProductBaseCode=SL
  Mux : Mux  Inputs=2
  Out1 : Outport
  wires:
  Bit Slice/1 -> Mux/1
  u/1 -> Bit Slice/1, Bit Slice1/1
  Bit Slice1/1 -> Mux/2
  Mux/1 -> Out1/1

== system ARAI_Academy/Subsystem13/Subsystem/Subsystem3 ==
  u : Inport
  Bit Slice : hdlsllib/Logic and Bit Operations/Bit Slice  lidx=15  ridx=8
      settings: SourceProductBaseCode=SL
  Bit Slice1 : hdlsllib/Logic and Bit Operations/Bit Slice  lidx=7  ridx=0
      settings: SourceProductBaseCode=SL
  Mux : Mux  Inputs=2
  Out1 : Outport
  wires:
  Bit Slice/1 -> Mux/1
  u/1 -> Bit Slice/1, Bit Slice1/1
  Bit Slice1/1 -> Mux/2
  Mux/1 -> Out1/1

== system ARAI_Academy/Subsystem13/Subsystem/Subsystem4 ==
  u : Inport
  Bit Slice : hdlsllib/Logic and Bit Operations/Bit Slice  lidx=15  ridx=8
      settings: SourceProductBaseCode=SL
  Bit Slice1 : hdlsllib/Logic and Bit Operations/Bit Slice  lidx=7  ridx=0
      settings: SourceProductBaseCode=SL
  Mux : Mux  Inputs=2
  Out1 : Outport
  wires:
  Bit Slice/1 -> Mux/1
  u/1 -> Bit Slice/1, Bit Slice1/1
  Bit Slice1/1 -> Mux/2
  Mux/1 -> Out1/1

== system ARAI_Academy/Subsystem13/Subsystem/Subsystem5 ==
  u : Inport
  Bit Slice : hdlsllib/Logic and Bit Operations/Bit Slice  lidx=15  ridx=8
      settings: SourceProductBaseCode=SL
  Bit Slice1 : hdlsllib/Logic and Bit Operations/Bit Slice  lidx=7  ridx=0
      settings: SourceProductBaseCode=SL
  Mux : Mux  Inputs=2
  Out1 : Outport
  wires:
  Bit Slice/1 -> Mux/1
  u/1 -> Bit Slice/1, Bit Slice1/1
  Bit Slice1/1 -> Mux/2
  Mux/1 -> Out1/1

== system ARAI_Academy/Subsystem13/Subsystem/Subsystem6 ==
  u : Inport
  Bit Slice : hdlsllib/Logic and Bit Operations/Bit Slice  lidx=15  ridx=8
      settings: SourceProductBaseCode=SL
  Bit Slice1 : hdlsllib/Logic and Bit Operations/Bit Slice  lidx=7  ridx=0
      settings: SourceProductBaseCode=SL
  Mux : Mux  Inputs=2
  Out1 : Outport
  wires:
  Bit Slice/1 -> Mux/1
  u/1 -> Bit Slice/1, Bit Slice1/1
  Bit Slice1/1 -> Mux/2
  Mux/1 -> Out1/1

== system ARAI_Academy/Subsystem13/Subsystem/Subsystem7 ==
  u : Inport
  Bit Slice : hdlsllib/Logic and Bit Operations/Bit Slice  lidx=15  ridx=8
      settings: SourceProductBaseCode=SL
  Bit Slice1 : hdlsllib/Logic and Bit Operations/Bit Slice  lidx=7  ridx=0
      settings: SourceProductBaseCode=SL
  Mux : Mux  Inputs=2
  Out1 : Outport
  wires:
  Mux/1 -> Out1/1
  Bit Slice1/1 -> Mux/2
  u/1 -> Bit Slice1/1, Bit Slice/1
  Bit Slice/1 -> Mux/1

== system ARAI_Academy/Subsystem13/Subsystem/Subsystem8 ==
  u : Inport
  Bit Slice : hdlsllib/Logic and Bit Operations/Bit Slice  lidx=15  ridx=8
      settings: SourceProductBaseCode=SL
  Bit Slice1 : hdlsllib/Logic and Bit Operations/Bit Slice  lidx=7  ridx=0
      settings: SourceProductBaseCode=SL
  Mux : Mux  Inputs=2
  Out1 : Outport
  wires:
  Bit Slice/1 -> Mux/1
  u/1 -> Bit Slice/1, Bit Slice1/1
  Bit Slice1/1 -> Mux/2
  Mux/1 -> Out1/1

== system ARAI_Academy/Subsystem13/Subsystem/Subsystem9 ==
  u : Inport
  Bit Slice : hdlsllib/Logic and Bit Operations/Bit Slice  lidx=15  ridx=8
      settings: SourceProductBaseCode=SL
  Bit Slice1 : hdlsllib/Logic and Bit Operations/Bit Slice  lidx=7  ridx=0
      settings: SourceProductBaseCode=SL
  Mux : Mux  Inputs=2
  Out1 : Outport
  wires:
  Mux/1 -> Out1/1
  Bit Slice1/1 -> Mux/2
  u/1 -> Bit Slice1/1, Bit Slice/1
  Bit Slice/1 -> Mux/1

== system ARAI_Academy/Subsystem14/Subsystem/Subsystem ==
  u : Inport
  Bit Slice : hdlsllib/Logic and Bit Operations/Bit Slice  lidx=15  ridx=8
      settings: SourceProductBaseCode=SL
  Bit Slice1 : hdlsllib/Logic and Bit Operations/Bit Slice  lidx=7  ridx=0
      settings: SourceProductBaseCode=SL
  Mux : Mux  Inputs=2
  Out1 : Outport
  wires:
  Bit Slice/1 -> Mux/1
  u/1 -> Bit Slice/1, Bit Slice1/1
  Bit Slice1/1 -> Mux/2
  Mux/1 -> Out1/1

== system ARAI_Academy/Subsystem14/Subsystem/Subsystem1 ==
  u : Inport
  Bit Slice : hdlsllib/Logic and Bit Operations/Bit Slice  lidx=15  ridx=8
      settings: SourceProductBaseCode=SL
  Bit Slice1 : hdlsllib/Logic and Bit Operations/Bit Slice  lidx=7  ridx=0
      settings: SourceProductBaseCode=SL
  Mux : Mux  Inputs=2
  Out1 : Outport
  wires:
  Bit Slice/1 -> Mux/1
  u/1 -> Bit Slice/1, Bit Slice1/1
  Bit Slice1/1 -> Mux/2
  Mux/1 -> Out1/1

== system ARAI_Academy/Subsystem14/Subsystem/Subsystem10 ==
  u : Inport
  Bit Slice : hdlsllib/Logic and Bit Operations/Bit Slice  lidx=15  ridx=8
      settings: SourceProductBaseCode=SL
  Bit Slice1 : hdlsllib/Logic and Bit Operations/Bit Slice  lidx=7  ridx=0
      settings: SourceProductBaseCode=SL
  Mux : Mux  Inputs=2
  Out1 : Outport
  wires:
  Bit Slice/1 -> Mux/1
  u/1 -> Bit Slice/1, Bit Slice1/1
  Bit Slice1/1 -> Mux/2
  Mux/1 -> Out1/1

== system ARAI_Academy/Subsystem14/Subsystem/Subsystem11 ==
  u : Inport
  Bit Slice : hdlsllib/Logic and Bit Operations/Bit Slice  lidx=15  ridx=8
      settings: SourceProductBaseCode=SL
  Bit Slice1 : hdlsllib/Logic and Bit Operations/Bit Slice  lidx=7  ridx=0
      settings: SourceProductBaseCode=SL
  Mux : Mux  Inputs=2
  Out1 : Outport
  wires:
  Mux/1 -> Out1/1
  Bit Slice1/1 -> Mux/2
  u/1 -> Bit Slice1/1, Bit Slice/1
  Bit Slice/1 -> Mux/1

== system ARAI_Academy/Subsystem14/Subsystem/Subsystem12 ==
  u : Inport
  Bit Slice : hdlsllib/Logic and Bit Operations/Bit Slice  lidx=15  ridx=8
      settings: SourceProductBaseCode=SL
  Bit Slice1 : hdlsllib/Logic and Bit Operations/Bit Slice  lidx=7  ridx=0
      settings: SourceProductBaseCode=SL
  Mux : Mux  Inputs=2
  Out1 : Outport
  wires:
  Bit Slice/1 -> Mux/1
  u/1 -> Bit Slice/1, Bit Slice1/1
  Bit Slice1/1 -> Mux/2
  Mux/1 -> Out1/1

== system ARAI_Academy/Subsystem14/Subsystem/Subsystem13 ==
  u : Inport
  Bit Slice : hdlsllib/Logic and Bit Operations/Bit Slice  lidx=15  ridx=8
      settings: SourceProductBaseCode=SL
  Bit Slice1 : hdlsllib/Logic and Bit Operations/Bit Slice  lidx=7  ridx=0
      settings: SourceProductBaseCode=SL
  Mux : Mux  Inputs=2
  Out1 : Outport
  wires:
  Mux/1 -> Out1/1
  Bit Slice1/1 -> Mux/2
  u/1 -> Bit Slice1/1, Bit Slice/1
  Bit Slice/1 -> Mux/1

== system ARAI_Academy/Subsystem14/Subsystem/Subsystem14 ==
  u : Inport
  Bit Slice : hdlsllib/Logic and Bit Operations/Bit Slice  lidx=15  ridx=8
      settings: SourceProductBaseCode=SL
  Bit Slice1 : hdlsllib/Logic and Bit Operations/Bit Slice  lidx=7  ridx=0
      settings: SourceProductBaseCode=SL
  Mux : Mux  Inputs=2
  Out1 : Outport
  wires:
  Bit Slice/1 -> Mux/1
  u/1 -> Bit Slice/1, Bit Slice1/1
  Bit Slice1/1 -> Mux/2
  Mux/1 -> Out1/1

== system ARAI_Academy/Subsystem14/Subsystem/Subsystem15 ==
  u : Inport
  Bit Slice : hdlsllib/Logic and Bit Operations/Bit Slice  lidx=15  ridx=8
      settings: SourceProductBaseCode=SL
  Bit Slice1 : hdlsllib/Logic and Bit Operations/Bit Slice  lidx=7  ridx=0
      settings: SourceProductBaseCode=SL
  Mux : Mux  Inputs=2
  Out1 : Outport
  wires:
  Mux/1 -> Out1/1
  Bit Slice1/1 -> Mux/2
  u/1 -> Bit Slice1/1, Bit Slice/1
  Bit Slice/1 -> Mux/1

== system ARAI_Academy/Subsystem14/Subsystem/Subsystem2 ==
  u : Inport
  Bit Slice : hdlsllib/Logic and Bit Operations/Bit Slice  lidx=15  ridx=8
      settings: SourceProductBaseCode=SL
  Bit Slice1 : hdlsllib/Logic and Bit Operations/Bit Slice  lidx=7  ridx=0
      settings: SourceProductBaseCode=SL
  Mux : Mux  Inputs=2
  Out1 : Outport
  wires:
  Bit Slice/1 -> Mux/1
  u/1 -> Bit Slice/1, Bit Slice1/1
  Bit Slice1/1 -> Mux/2
  Mux/1 -> Out1/1

== system ARAI_Academy/Subsystem14/Subsystem/Subsystem3 ==
  u : Inport
  Bit Slice : hdlsllib/Logic and Bit Operations/Bit Slice  lidx=15  ridx=8
      settings: SourceProductBaseCode=SL
  Bit Slice1 : hdlsllib/Logic and Bit Operations/Bit Slice  lidx=7  ridx=0
      settings: SourceProductBaseCode=SL
  Mux : Mux  Inputs=2
  Out1 : Outport
  wires:
  Bit Slice/1 -> Mux/1
  u/1 -> Bit Slice/1, Bit Slice1/1
  Bit Slice1/1 -> Mux/2
  Mux/1 -> Out1/1

== system ARAI_Academy/Subsystem14/Subsystem/Subsystem4 ==
  u : Inport
  Bit Slice : hdlsllib/Logic and Bit Operations/Bit Slice  lidx=15  ridx=8
      settings: SourceProductBaseCode=SL
  Bit Slice1 : hdlsllib/Logic and Bit Operations/Bit Slice  lidx=7  ridx=0
      settings: SourceProductBaseCode=SL
  Mux : Mux  Inputs=2
  Out1 : Outport
  wires:
  Bit Slice/1 -> Mux/1
  u/1 -> Bit Slice/1, Bit Slice1/1
  Bit Slice1/1 -> Mux/2
  Mux/1 -> Out1/1

== system ARAI_Academy/Subsystem14/Subsystem/Subsystem5 ==
  u : Inport
  Bit Slice : hdlsllib/Logic and Bit Operations/Bit Slice  lidx=15  ridx=8
      settings: SourceProductBaseCode=SL
  Bit Slice1 : hdlsllib/Logic and Bit Operations/Bit Slice  lidx=7  ridx=0
      settings: SourceProductBaseCode=SL
  Mux : Mux  Inputs=2
  Out1 : Outport
  wires:
  Bit Slice/1 -> Mux/1
  u/1 -> Bit Slice/1, Bit Slice1/1
  Bit Slice1/1 -> Mux/2
  Mux/1 -> Out1/1

== system ARAI_Academy/Subsystem14/Subsystem/Subsystem6 ==
  u : Inport
  Bit Slice : hdlsllib/Logic and Bit Operations/Bit Slice  lidx=15  ridx=8
      settings: SourceProductBaseCode=SL
  Bit Slice1 : hdlsllib/Logic and Bit Operations/Bit Slice  lidx=7  ridx=0
      settings: SourceProductBaseCode=SL
  Mux : Mux  Inputs=2
  Out1 : Outport
  wires:
  Bit Slice/1 -> Mux/1
  u/1 -> Bit Slice/1, Bit Slice1/1
  Bit Slice1/1 -> Mux/2
  Mux/1 -> Out1/1

== system ARAI_Academy/Subsystem14/Subsystem/Subsystem7 ==
  u : Inport
  Bit Slice : hdlsllib/Logic and Bit Operations/Bit Slice  lidx=15  ridx=8
      settings: SourceProductBaseCode=SL
  Bit Slice1 : hdlsllib/Logic and Bit Operations/Bit Slice  lidx=7  ridx=0
      settings: SourceProductBaseCode=SL
  Mux : Mux  Inputs=2
  Out1 : Outport
  wires:
  Mux/1 -> Out1/1
  Bit Slice1/1 -> Mux/2
  u/1 -> Bit Slice1/1, Bit Slice/1
  Bit Slice/1 -> Mux/1

== system ARAI_Academy/Subsystem14/Subsystem/Subsystem8 ==
  u : Inport
  Bit Slice : hdlsllib/Logic and Bit Operations/Bit Slice  lidx=15  ridx=8
      settings: SourceProductBaseCode=SL
  Bit Slice1 : hdlsllib/Logic and Bit Operations/Bit Slice  lidx=7  ridx=0
      settings: SourceProductBaseCode=SL
  Mux : Mux  Inputs=2
  Out1 : Outport
  wires:
  Bit Slice/1 -> Mux/1
  u/1 -> Bit Slice/1, Bit Slice1/1
  Bit Slice1/1 -> Mux/2
  Mux/1 -> Out1/1

== system ARAI_Academy/Subsystem14/Subsystem/Subsystem9 ==
  u : Inport
  Bit Slice : hdlsllib/Logic and Bit Operations/Bit Slice  lidx=15  ridx=8
      settings: SourceProductBaseCode=SL
  Bit Slice1 : hdlsllib/Logic and Bit Operations/Bit Slice  lidx=7  ridx=0
      settings: SourceProductBaseCode=SL
  Mux : Mux  Inputs=2
  Out1 : Outport
  wires:
  Mux/1 -> Out1/1
  Bit Slice1/1 -> Mux/2
  u/1 -> Bit Slice1/1, Bit Slice/1
  Bit Slice/1 -> Mux/1

== system ARAI_Academy/Subsystem14/Subsystem8/Subsystem ==
  u : Inport
  Bit Slice : hdlsllib/Logic and Bit Operations/Bit Slice  lidx=15  ridx=8
      settings: SourceProductBaseCode=SL
  Bit Slice1 : hdlsllib/Logic and Bit Operations/Bit Slice  lidx=7  ridx=0
      settings: SourceProductBaseCode=SL
  Mux : Mux  Inputs=2
  Out1 : Outport
  wires:
  Bit Slice/1 -> Mux/1
  u/1 -> Bit Slice/1, Bit Slice1/1
  Bit Slice1/1 -> Mux/2
  Mux/1 -> Out1/1

== system ARAI_Academy/Subsystem14/Subsystem8/Subsystem1 ==
  u : Inport
  Bit Slice : hdlsllib/Logic and Bit Operations/Bit Slice  lidx=15  ridx=8
      settings: SourceProductBaseCode=SL
  Bit Slice1 : hdlsllib/Logic and Bit Operations/Bit Slice  lidx=7  ridx=0
      settings: SourceProductBaseCode=SL
  Mux : Mux  Inputs=2
  Out1 : Outport
  wires:
  Bit Slice/1 -> Mux/1
  u/1 -> Bit Slice/1, Bit Slice1/1
  Bit Slice1/1 -> Mux/2
  Mux/1 -> Out1/1

== system ARAI_Academy/Subsystem14/Subsystem8/Subsystem2 ==
  u : Inport
  Bit Slice : hdlsllib/Logic and Bit Operations/Bit Slice  lidx=15  ridx=8
      settings: SourceProductBaseCode=SL
  Bit Slice1 : hdlsllib/Logic and Bit Operations/Bit Slice  lidx=7  ridx=0
      settings: SourceProductBaseCode=SL
  Mux : Mux  Inputs=2
  Out1 : Outport
  wires:
  Bit Slice/1 -> Mux/1
  u/1 -> Bit Slice/1, Bit Slice1/1
  Bit Slice1/1 -> Mux/2
  Mux/1 -> Out1/1

== system ARAI_Academy/Subsystem14/Subsystem8/Subsystem3 ==
  u : Inport
  Bit Slice : hdlsllib/Logic and Bit Operations/Bit Slice  lidx=15  ridx=8
      settings: SourceProductBaseCode=SL
  Bit Slice1 : hdlsllib/Logic and Bit Operations/Bit Slice  lidx=7  ridx=0
      settings: SourceProductBaseCode=SL
  Mux : Mux  Inputs=2
  Out1 : Outport
  wires:
  Bit Slice/1 -> Mux/1
  u/1 -> Bit Slice/1, Bit Slice1/1
  Bit Slice1/1 -> Mux/2
  Mux/1 -> Out1/1

== system ARAI_Academy/Subsystem14/Subsystem8/Subsystem4 ==
  u : Inport
  Bit Slice : hdlsllib/Logic and Bit Operations/Bit Slice  lidx=15  ridx=8
      settings: SourceProductBaseCode=SL
  Bit Slice1 : hdlsllib/Logic and Bit Operations/Bit Slice  lidx=7  ridx=0
      settings: SourceProductBaseCode=SL
  Mux : Mux  Inputs=2
  Out1 : Outport
  wires:
  Bit Slice/1 -> Mux/1
  u/1 -> Bit Slice/1, Bit Slice1/1
  Bit Slice1/1 -> Mux/2
  Mux/1 -> Out1/1

== system ARAI_Academy/Subsystem14/Subsystem8/Subsystem5 ==
  u : Inport
  Bit Slice : hdlsllib/Logic and Bit Operations/Bit Slice  lidx=15  ridx=8
      settings: SourceProductBaseCode=SL
  Bit Slice1 : hdlsllib/Logic and Bit Operations/Bit Slice  lidx=7  ridx=0
      settings: SourceProductBaseCode=SL
  Mux : Mux  Inputs=2
  Out1 : Outport
  wires:
  Bit Slice/1 -> Mux/1
  u/1 -> Bit Slice/1, Bit Slice1/1
  Bit Slice1/1 -> Mux/2
  Mux/1 -> Out1/1

== system ARAI_Academy/Subsystem14/Subsystem8/Subsystem7 ==
  u : Inport
  Bit Slice : hdlsllib/Logic and Bit Operations/Bit Slice  lidx=15  ridx=8
      settings: SourceProductBaseCode=SL
  Bit Slice1 : hdlsllib/Logic and Bit Operations/Bit Slice  lidx=7  ridx=0
      settings: SourceProductBaseCode=SL
  Mux : Mux  Inputs=2
  Out1 : Outport
  wires:
  Mux/1 -> Out1/1
  Bit Slice1/1 -> Mux/2
  u/1 -> Bit Slice1/1, Bit Slice/1
  Bit Slice/1 -> Mux/1

== system ARAI_Academy/Subsystem14/Subsystem8/Subsystem8 ==
  u : Inport
  Bit Slice : hdlsllib/Logic and Bit Operations/Bit Slice  lidx=15  ridx=8
      settings: SourceProductBaseCode=SL
  Bit Slice1 : hdlsllib/Logic and Bit Operations/Bit Slice  lidx=7  ridx=0
      settings: SourceProductBaseCode=SL
  Mux : Mux  Inputs=2
  Out1 : Outport
  wires:
  Bit Slice/1 -> Mux/1
  u/1 -> Bit Slice/1, Bit Slice1/1
  Bit Slice1/1 -> Mux/2
  Mux/1 -> Out1/1

== system ARAI_Academy/Subsystem15/Subsystem12/Subsystem ==
  u : Inport
  Bit Slice : hdlsllib/Logic and Bit Operations/Bit Slice  lidx=15  ridx=8
      settings: SourceProductBaseCode=SL
  Bit Slice1 : hdlsllib/Logic and Bit Operations/Bit Slice  lidx=7  ridx=0
      settings: SourceProductBaseCode=SL
  Mux : Mux  Inputs=2
  Out1 : Outport
  wires:
  Bit Slice/1 -> Mux/1
  u/1 -> Bit Slice/1, Bit Slice1/1
  Bit Slice1/1 -> Mux/2
  Mux/1 -> Out1/1

== system ARAI_Academy/Subsystem15/Subsystem12/Subsystem1 ==
  u : Inport
  Bit Slice : hdlsllib/Logic and Bit Operations/Bit Slice  lidx=15  ridx=8
      settings: SourceProductBaseCode=SL
  Bit Slice1 : hdlsllib/Logic and Bit Operations/Bit Slice  lidx=7  ridx=0
      settings: SourceProductBaseCode=SL
  Mux : Mux  Inputs=2
  Out1 : Outport
  wires:
  Bit Slice/1 -> Mux/1
  u/1 -> Bit Slice/1, Bit Slice1/1
  Bit Slice1/1 -> Mux/2
  Mux/1 -> Out1/1

== system ARAI_Academy/Subsystem15/Subsystem12/Subsystem2 ==
  u : Inport
  Bit Slice : hdlsllib/Logic and Bit Operations/Bit Slice  lidx=15  ridx=8
      settings: SourceProductBaseCode=SL
  Bit Slice1 : hdlsllib/Logic and Bit Operations/Bit Slice  lidx=7  ridx=0
      settings: SourceProductBaseCode=SL
  Mux : Mux  Inputs=2
  Out1 : Outport
  wires:
  Bit Slice/1 -> Mux/1
  u/1 -> Bit Slice/1, Bit Slice1/1
  Bit Slice1/1 -> Mux/2
  Mux/1 -> Out1/1

== system ARAI_Academy/Subsystem15/Subsystem12/Subsystem3 ==
  u : Inport
  Bit Slice : hdlsllib/Logic and Bit Operations/Bit Slice  lidx=15  ridx=8
      settings: SourceProductBaseCode=SL
  Bit Slice1 : hdlsllib/Logic and Bit Operations/Bit Slice  lidx=7  ridx=0
      settings: SourceProductBaseCode=SL
  Mux : Mux  Inputs=2
  Out1 : Outport
  wires:
  Bit Slice/1 -> Mux/1
  u/1 -> Bit Slice/1, Bit Slice1/1
  Bit Slice1/1 -> Mux/2
  Mux/1 -> Out1/1

== system ARAI_Academy/Subsystem15/Subsystem12/Subsystem4 ==
  u : Inport
  Bit Slice : hdlsllib/Logic and Bit Operations/Bit Slice  lidx=15  ridx=8
      settings: SourceProductBaseCode=SL
  Bit Slice1 : hdlsllib/Logic and Bit Operations/Bit Slice  lidx=7  ridx=0
      settings: SourceProductBaseCode=SL
  Mux : Mux  Inputs=2
  Out1 : Outport
  wires:
  Bit Slice/1 -> Mux/1
  u/1 -> Bit Slice/1, Bit Slice1/1
  Bit Slice1/1 -> Mux/2
  Mux/1 -> Out1/1

== system ARAI_Academy/Subsystem15/Subsystem12/Subsystem5 ==
  u : Inport
  Bit Slice : hdlsllib/Logic and Bit Operations/Bit Slice  lidx=15  ridx=8
      settings: SourceProductBaseCode=SL
  Bit Slice1 : hdlsllib/Logic and Bit Operations/Bit Slice  lidx=7  ridx=0
      settings: SourceProductBaseCode=SL
  Mux : Mux  Inputs=2
  Out1 : Outport
  wires:
  Bit Slice/1 -> Mux/1
  u/1 -> Bit Slice/1, Bit Slice1/1
  Bit Slice1/1 -> Mux/2
  Mux/1 -> Out1/1

== system ARAI_Academy/Subsystem15/Subsystem12/Subsystem7 ==
  u : Inport
  Bit Slice : hdlsllib/Logic and Bit Operations/Bit Slice  lidx=15  ridx=8
      settings: SourceProductBaseCode=SL
  Bit Slice1 : hdlsllib/Logic and Bit Operations/Bit Slice  lidx=7  ridx=0
      settings: SourceProductBaseCode=SL
  Mux : Mux  Inputs=2
  Out1 : Outport
  wires:
  Mux/1 -> Out1/1
  Bit Slice1/1 -> Mux/2
  u/1 -> Bit Slice1/1, Bit Slice/1
  Bit Slice/1 -> Mux/1
